simulink model "Rigid_1DOF_kinematics"  (R2020b)
settings: Solver=VariableStepAuto  StartTime=0.0  StopTime=10.0  RelTol=1e-3
libraries: vrlib x2
settings Model: Creator=beave  LastModifiedBy=beave

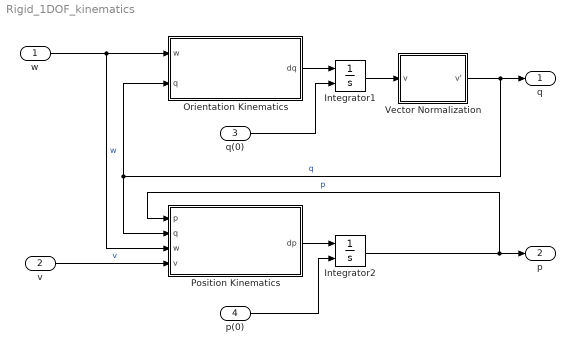
== system Rigid_1DOF_kinematics ==
  w : Inport  PortDimensions=3
  v : Inport  Port=2  PortDimensions=3
  q(0) : Inport  Port=3  PortDimensions=4
  p(0) : Inport  Port=4  PortDimensions=3
  Integrator1 : Integrator  InitialConditionSource=external
  Integrator2 : Integrator  InitialConditionSource=external
  Orientation Kinematics : Subsystem
  Position Kinematics : Subsystem
  Vector Normalization : Subsystem
      mask Display: disp('v''=v/|v|')
  q : Outport
  p : Outport  Port=2
  wires:
  q(0)/1 -> Integrator1/2
  w/1 -> Position Kinematics/3(w), Orientation Kinematics/1(w)  "w"
  Orientation Kinematics/1(dq) -> Integrator1/1
  Integrator1/1 -> Vector Normalization/1(v)
  Vector Normalization/1(v') -> q/1, Position Kinematics/2(q), Orientation Kinematics/2(q)  "q"
  Position Kinematics/1(dp) -> Integrator2/1
  Integrator2/1 -> p/1, Position Kinematics/1(p)  "p"
  p(0)/1 -> Integrator2/2
  v/1 -> Position Kinematics/4(v)  "v"

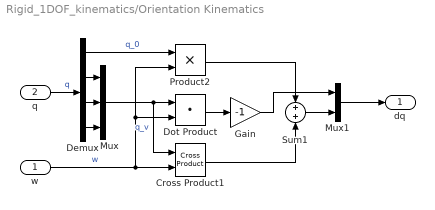
== system Rigid_1DOF_kinematics/Orientation Kinematics ==
  w : Inport
  q : Inport  Port=2
  Cross Product1 : vrlib/Utilities/Cross Product
  Demux : Demux
  Dot Product : DotProduct  InputSameDT=on  OutDataTypeStr=Inherit: Inherit via internal rule
  Gain : Gain  Gain=-1
  Mux : Mux  Inputs=3
  Mux1 : Mux  Inputs=2
  Product2 : Product
  Sum1 : Sum  Inputs=+|+
  dq : Outport
  wires:
  q/1 -> Demux/1  "q"
  Sum1/1 -> Mux1/2
  Gain/1 -> Mux1/1
  Demux/2 -> Mux/1
  Demux/3 -> Mux/2
  Cross Product1/1 -> Sum1/2
  w/1 -> Cross Product1/2, Product2/2, Dot Product/2  "w"
  Demux/4 -> Mux/3
  Mux/1 -> Cross Product1/1, Dot Product/1  "q_v"
  Demux/1 -> Product2/1  "q_0"
  Dot Product/1 -> Gain/1
  Product2/1 -> Sum1/1
  Mux1/1 -> dq/1

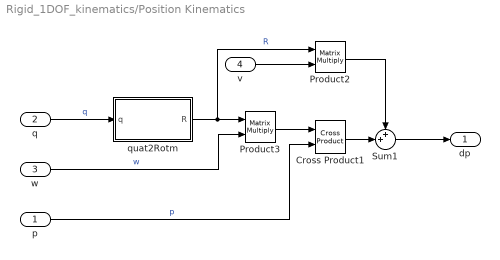
== system Rigid_1DOF_kinematics/Position Kinematics ==
  p : Inport
  q : Inport  Port=2
  w : Inport  Port=3
  v : Inport  Port=4
  Cross Product1 : vrlib/Utilities/Cross Product
  Product2 : Product  Multiplication=Matrix(*)
  Product3 : Product  Multiplication=Matrix(*)
  Sum1 : Sum  Inputs=++|
  quat2Rotm : Subsystem
      mask Display: disp('R(q)')
  dp : Outport
  wires:
  w/1 -> Product3/2  "w"
  quat2Rotm/1(R) -> Product2/1, Product3/1  "R"
  Sum1/1 -> dp/1
  q/1 -> quat2Rotm/1(q)  "q"
  Product3/1 -> Cross Product1/1
  Product2/1 -> Sum1/1
  p/1 -> Cross Product1/2  "p"
  Cross Product1/1 -> Sum1/2
  v/1 -> Product2/2

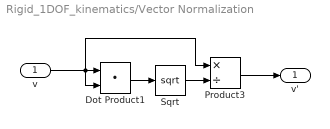
== system Rigid_1DOF_kinematics/Vector Normalization ==
  v : Inport
  Dot Product1 : DotProduct  InputSameDT=on  OutDataTypeStr=Inherit: Inherit via internal rule
  Product3 : Product  Inputs=*/
  Sqrt : Sqrt  SaturateOnIntegerOverflow=on
  v' : Outport
  wires:
  Product3/1 -> v'/1
  v/1 -> Dot Product1/2, Product3/1, Dot Product1/1
  Dot Product1/1 -> Sqrt/1
  Sqrt/1 -> Product3/2

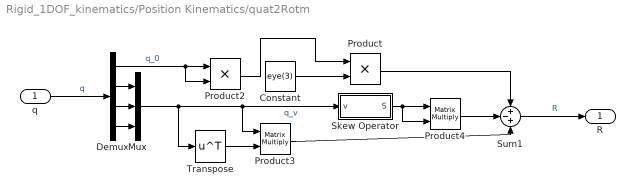
== system Rigid_1DOF_kinematics/Position Kinematics/quat2Rotm ==
  q : Inport
  Constant : Constant  Value=eye(3)
  Demux : Demux
  Mux : Mux  Inputs=3
  Product : Product
  Product2 : Product
  Product3 : Product  Multiplication=Matrix(*)
  Product4 : Product  Multiplication=Matrix(*)
  Skew Operator : Subsystem  Description=S(v)
      mask Display: disp('S(v)')
  Sum1 : Sum  Inputs=+-+
  Transpose : Math  Operator=transpose  SaturateOnIntegerOverflow=on
  R : Outport
  wires:
  q/1 -> Demux/1  "q"
  Sum1/1 -> R/1  "R"
  Mux/1 -> Transpose/1, Product3/1, Skew Operator/1(v)  "q_v"
  Skew Operator/1(S) -> Product4/2, Product4/1
  Demux/1 -> Product2/2, Product2/1  "q_0"
  Product2/1 -> Product/1
  Transpose/1 -> Product3/2
  Product/1 -> Sum1/1
  Demux/2 -> Mux/1
  Product3/1 -> Sum1/3
  Demux/3 -> Mux/2
  Demux/4 -> Mux/3
  Product4/1 -> Sum1/2
  Constant/1 -> Product/2

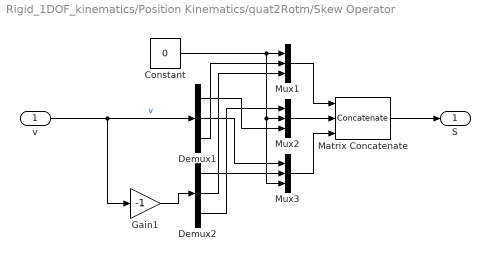
== system Rigid_1DOF_kinematics/Position Kinematics/quat2Rotm/Skew Operator ==
  v : Inport
  Constant : Constant  Value=0
  Demux1 : Demux  Outputs=3
  Demux2 : Demux  Outputs=3
  Gain1 : Gain  Gain=-1
  Matrix Concatenate : Concatenate  NumInputs=3  Mode=Multidimensional array  ConcatenateDimension=2
  Mux1 : Mux  Inputs=3
  Mux2 : Mux  Inputs=3
  Mux3 : Mux  Inputs=3
  S : Outport
  wires:
  Constant/1 -> Mux3/3, Mux2/2, Mux1/1
  Demux1/3 -> Mux1/2
  Matrix Concatenate/1 -> S/1
  Demux1/1 -> Mux2/3
  v/1 -> Demux1/1, Gain1/1  "v"
  Demux2/1 -> Mux3/2
  Mux3/1 -> Matrix Concatenate/3
  Gain1/1 -> Demux2/1
  Demux2/3 -> Mux2/1
  Mux1/1 -> Matrix Concatenate/1
  Demux2/2 -> Mux1/3
  Demux1/2 -> Mux3/1
  Mux2/1 -> Matrix Concatenate/2
